simulink model "UR5_simulink"  (R2022b)
settings: Solver=FixedStepAuto  StartTime=0.0  StopTime=8  FixedStep=1e-4  RelTol=1e-3  AbsTol=1e-3  EnableMultiTasking=on
values from neighbouring files (symbols this model uses):
  a1 = 0    [UR5_matlab.m]
  a2 = -0.425    [UR5_matlab.m]
  a3 = -0.39225    [UR5_matlab.m]
  a4 = 0    [UR5_matlab.m]
  a5 = 0    [UR5_matlab.m]
  a6 = 0    [UR5_matlab.m]
  d1 = 0.089159    [UR5_matlab.m]
  d2 = 0    [UR5_matlab.m]
  d3 = 0    [UR5_matlab.m]
  d4 = 0.10915    [UR5_matlab.m]
  d5 = 0.09465    [UR5_matlab.m]
  d6 = 0.0823    [UR5_matlab.m]
  K_fb_1 = fb_action(K1_20,N,Jin_20,Bmw,J1_est,wR1)    [UR5_matlab.m]
  K_fb_2 = fb_action(K1_20,N,Jin_20,Bmw,J2_est,wR2)    [UR5_matlab.m]
  K_fb_3 = fb_action(K1_20,N,Jin_20,Bmw,J3_est,wR3)    [UR5_matlab.m]
  K_fb_4 = fb_action(K1_14,N,Jin_14,Bmw,J4_est,wR4)    [UR5_matlab.m]
  K_fb_5 = fb_action(K1_14,N,Jin_14,Bmw,J5_est,wR5)    [UR5_matlab.m]
  K_fb_6 = fb_action(K1_14,N,Jin_14,Bmw,J6_est,wR6)    [UR5_matlab.m]
  m1 = 3.7    [UR5_matlab.m]
  m2 = 8.393    [UR5_matlab.m]
  m3 = 2.33    [UR5_matlab.m]
  m4 = 1.1219    [UR5_matlab.m]
  m5 = 1.1219    [UR5_matlab.m]
  m6 = 0.1879    [UR5_matlab.m]
  N = 100    [UR5_matlab.m]
undefined symbols (not defined in the file or in its folder): X, Y, Z
libraries: fl_lib x60, sm_lib x33, nesl_utility x31, MyComponent_lib x12
(part 1 of 2)
settings Model: Creator=FrePa  LastModifiedBy=jacop
settings SolverCC: AutoScaleAbsTol=off  AlgebraicLoopSolver=TrustRegion
settings DebuggingCC: UnconnectedInputMsg=warning  UnconnectedOutputMsg=warning  UnconnectedLineMsg=warning  SymbolicDimsDataTypeCodeGenerationDiagnostic=none  SFMachineParentedDataDiag=warning
settings ModelReferenceCC: EnableRefExpFcnMdlSchedulingChecks=on
settings SFSimCC: CustomCodeUndefinedFunction=UseInterfaceOnly
settings RTWCC: DLArmComputeVersion=19.05
settings SimscapeCC: SimscapeLogType=all  SimscapeLogSimulationStatistics=on  SimscapeLogDataHistory=10000
settings ExplorerConfigSet: InternalSimMechanicsExplorerSettings="<ExplorerConfiguration><canonicalview>default</canonicalview><AnimationSetting><BasePlaybackSpeed>1.0</BasePlaybackSpeed><PlaybackSpeedFactor>1.0</PlaybackSpeedFactor></AnimationSetting><TilePanel><TileInfo><Tiles Columns=\"1\" Count=\"1\" Rows=\"1\"><Column Weight=\"1\"/><Row Weight=\"1\"/><Tile Height=\"1\" Width=\"1\" X=\"0\" Y=\"0\"/></Tiles></TileInfo><SceneInfo><SceneViewer><BGColor><R>0.800000011920928955</R><G>0.800000011920928955</G><B>0.800000011920928955</B></BGColor><Camera><DoPerspective>off</DoPerspective><Position><X>-0.833530405890455017</X><Y>-1.17623602270469418</Y><Z>0.420539871522679465</Z></Position><Center><X>0.0136349575198428698</X><Y>0.0260154314115551427</Y><Z>0.247488077140803453</Z></Center><Up><X>0.101701536908081563</X><Y>0.0711627058760085085</Y><Z>0.992266429283455653</Z></Up><ViewLimDist>1</ViewLimDist><YLim>0.821541127691972517</YLim><XLim>1.22120978440698602</XLim></Camera></SceneViewer></SceneInfo></TilePanel><MechEditorPanel><Cameras/><GfxPanelCameraMap/><VideoCreator><PlaybackSpeedRatio>1.0</PlaybackSpeedRatio><FrameRate>30</FrameRate><VideoFormat>Motion JPEG AVI</VideoFormat><FrameSize>auto</FrameSize></VideoCreator></MechEditorPanel></ExplorerConfiguration>"

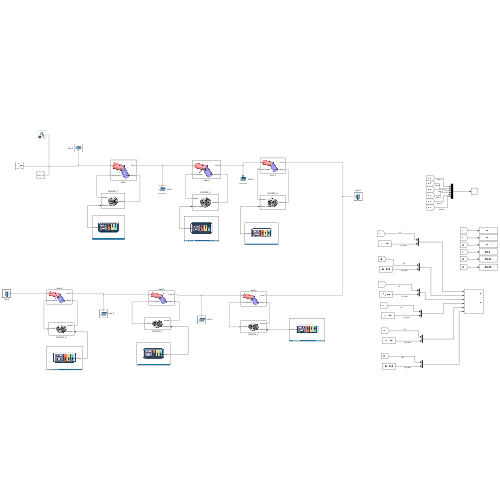
[thumbnail: Simulink's stored preview of the top-level diagram]
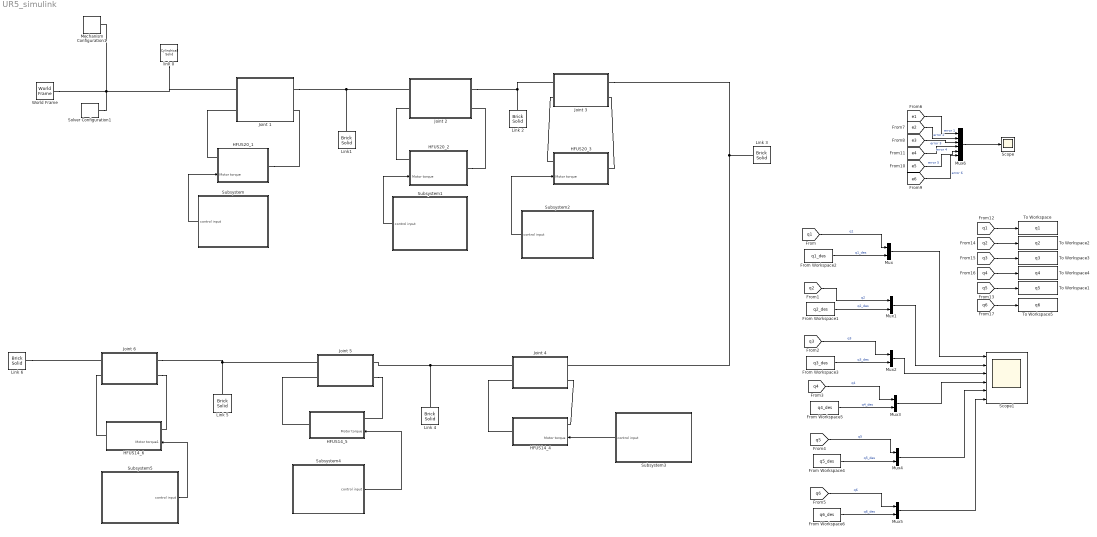
== system UR5_simulink ==
  From Workspace1 : FromWorkspace  VariableName=q2_des
  From Workspace2 : FromWorkspace  VariableName=q1_des
  From Workspace3 : FromWorkspace  VariableName=q3_des
  From Workspace4 : FromWorkspace  VariableName=q5_des
  From Workspace5 : FromWorkspace  VariableName=q4_des
  From Workspace6 : FromWorkspace  VariableName=q6_des
  HFUS14_4 : Subsystem
      settings: PortSchema="{\"entries\":[{\"content\":{\"sides\":[{\"content\":{\"connectorIds\":[\"LConn1\",\"In1\"]},\"type\":\"ConnectorPlacement.EquallySpacedRectSide\",\"uuid\":\"4949b501-9e24-4d03-87d2-659e8cd3beb4\"},{\"content\":{\"connectorIds\":[\"RConn1\"],\"side\":\"RIGHT\"},\"type\":\"ConnectorPlacement.EquallySpacedRectSide\",\"uuid\":\"cef4bc34-d56a-4a9d-a11a-d5ca4c8e0aed\"},{\"content\":{\"connectorIds\":[],\"side\":\"TOP\"},\"type\":\"ConnectorPlacement.EquallySpacedRectSide\",\"uuid\":\"8245fce7-f5cc-4776-a5c0-8930c8ed0033\"}]},\"type\":\"ConnectorPlacement.EquallySpacedConnector\",\"uuid\":\"b9012271-24e3-4605-81e2-55b4e9a8408d\"}],\"packageUris\":[\"http://schema.mathworks.com/mf0/Connector/R2020b\"],\"version\":\"1.0\"}"
      mask Display: image('images.jpeg'); % Use "Edit Image" on toolstrip to change.
  HFUS14_5 : Subsystem
      settings: PortSchema="{\"entries\":[{\"content\":{\"sides\":[{\"content\":{\"connectorIds\":[\"LConn1\",\"In1\"]},\"type\":\"ConnectorPlacement.EquallySpacedRectSide\",\"uuid\":\"4949b501-9e24-4d03-87d2-659e8cd3beb4\"},{\"content\":{\"connectorIds\":[\"RConn1\"],\"side\":\"RIGHT\"},\"type\":\"ConnectorPlacement.EquallySpacedRectSide\",\"uuid\":\"cef4bc34-d56a-4a9d-a11a-d5ca4c8e0aed\"},{\"content\":{\"connectorIds\":[],\"side\":\"TOP\"},\"type\":\"ConnectorPlacement.EquallySpacedRectSide\",\"uuid\":\"8245fce7-f5cc-4776-a5c0-8930c8ed0033\"}]},\"type\":\"ConnectorPlacement.EquallySpacedConnector\",\"uuid\":\"b9012271-24e3-4605-81e2-55b4e9a8408d\"}],\"packageUris\":[\"http://schema.mathworks.com/mf0/Connector/R2020b\"],\"version\":\"1.0\"}"
      mask Display: image('images.jpeg'); % Use "Edit Image" on toolstrip to change.
  HFUS14_6 : Subsystem
      settings: PortSchema="{\"entries\":[{\"content\":{\"sides\":[{\"content\":{\"connectorIds\":[\"LConn1\",\"In1\"]},\"type\":\"ConnectorPlacement.EquallySpacedRectSide\",\"uuid\":\"4949b501-9e24-4d03-87d2-659e8cd3beb4\"},{\"content\":{\"connectorIds\":[\"RConn1\"],\"side\":\"RIGHT\"},\"type\":\"ConnectorPlacement.EquallySpacedRectSide\",\"uuid\":\"cef4bc34-d56a-4a9d-a11a-d5ca4c8e0aed\"},{\"content\":{\"connectorIds\":[],\"side\":\"TOP\"},\"type\":\"ConnectorPlacement.EquallySpacedRectSide\",\"uuid\":\"8245fce7-f5cc-4776-a5c0-8930c8ed0033\"}]},\"type\":\"ConnectorPlacement.EquallySpacedConnector\",\"uuid\":\"b9012271-24e3-4605-81e2-55b4e9a8408d\"}],\"packageUris\":[\"http://schema.mathworks.com/mf0/Connector/R2020b\"],\"version\":\"1.0\"}"
      mask Display: image('images.jpeg'); % Use "Edit Image" on toolstrip to change.
  HFUS20_1 : Subsystem
      settings: PortSchema="{\"entries\":[{\"content\":{\"sides\":[{\"content\":{\"connectorIds\":[\"LConn1\",\"In1\"]},\"type\":\"ConnectorPlacement.EquallySpacedRectSide\",\"uuid\":\"4949b501-9e24-4d03-87d2-659e8cd3beb4\"},{\"content\":{\"connectorIds\":[\"RConn1\"],\"side\":\"RIGHT\"},\"type\":\"ConnectorPlacement.EquallySpacedRectSide\",\"uuid\":\"cef4bc34-d56a-4a9d-a11a-d5ca4c8e0aed\"},{\"content\":{\"connectorIds\":[],\"side\":\"TOP\"},\"type\":\"ConnectorPlacement.EquallySpacedRectSide\",\"uuid\":\"8245fce7-f5cc-4776-a5c0-8930c8ed0033\"}]},\"type\":\"ConnectorPlacement.EquallySpacedConnector\",\"uuid\":\"b9012271-24e3-4605-81e2-55b4e9a8408d\"}],\"packageUris\":[\"http://schema.mathworks.com/mf0/Connector/R2020b\"],\"version\":\"1.0\"}"
      mask Display: image('images.jpeg'); % Use "Edit Image" on toolstrip to change.
  HFUS20_2 : Subsystem
      settings: PortSchema="{\"entries\":[{\"content\":{\"sides\":[{\"content\":{\"connectorIds\":[\"LConn1\",\"In1\"]},\"type\":\"ConnectorPlacement.EquallySpacedRectSide\",\"uuid\":\"4949b501-9e24-4d03-87d2-659e8cd3beb4\"},{\"content\":{\"connectorIds\":[\"RConn1\"],\"side\":\"RIGHT\"},\"type\":\"ConnectorPlacement.EquallySpacedRectSide\",\"uuid\":\"cef4bc34-d56a-4a9d-a11a-d5ca4c8e0aed\"},{\"content\":{\"connectorIds\":[],\"side\":\"TOP\"},\"type\":\"ConnectorPlacement.EquallySpacedRectSide\",\"uuid\":\"8245fce7-f5cc-4776-a5c0-8930c8ed0033\"}]},\"type\":\"ConnectorPlacement.EquallySpacedConnector\",\"uuid\":\"b9012271-24e3-4605-81e2-55b4e9a8408d\"}],\"packageUris\":[\"http://schema.mathworks.com/mf0/Connector/R2020b\"],\"version\":\"1.0\"}"
      mask Display: image('images.jpeg'); % Use "Edit Image" on toolstrip to change.
  HFUS20_3 : Subsystem
      settings: PortSchema="{\"entries\":[{\"content\":{\"sides\":[{\"content\":{\"connectorIds\":[\"LConn1\",\"In1\"]},\"type\":\"ConnectorPlacement.EquallySpacedRectSide\",\"uuid\":\"4949b501-9e24-4d03-87d2-659e8cd3beb4\"},{\"content\":{\"connectorIds\":[\"RConn1\"],\"side\":\"RIGHT\"},\"type\":\"ConnectorPlacement.EquallySpacedRectSide\",\"uuid\":\"cef4bc34-d56a-4a9d-a11a-d5ca4c8e0aed\"},{\"content\":{\"connectorIds\":[],\"side\":\"TOP\"},\"type\":\"ConnectorPlacement.EquallySpacedRectSide\",\"uuid\":\"8245fce7-f5cc-4776-a5c0-8930c8ed0033\"}]},\"type\":\"ConnectorPlacement.EquallySpacedConnector\",\"uuid\":\"b9012271-24e3-4605-81e2-55b4e9a8408d\"}],\"packageUris\":[\"http://schema.mathworks.com/mf0/Connector/R2020b\"],\"version\":\"1.0\"}"
      mask Display: image('images.jpeg'); % Use "Edit Image" on toolstrip to change.
  Joint 1 : Subsystem
      mask Display: image('Revolute-1-DOF-Joint.png'); % Use "Edit Image" on toolstrip to change.
  Joint 2 : Subsystem
      mask Display: image('Revolute-1-DOF-Joint.png'); % Use "Edit Image" on toolstrip to change.
  Joint 3 : Subsystem
      mask Display: image('Revolute-1-DOF-Joint.png'); % Use "Edit Image" on toolstrip to change.
  Joint 4 : Subsystem
      mask Display: image('Revolute-1-DOF-Joint.png'); % Use "Edit Image" on toolstrip to change.
  Joint 5 : Subsystem
      mask Display: image('Revolute-1-DOF-Joint.png'); % Use "Edit Image" on toolstrip to change.
  Joint 6 : Subsystem
      mask Display: image('Revolute-1-DOF-Joint.png'); % Use "Edit Image" on toolstrip to change.
  Link 2 : sm_lib/Body Elements/Brick Solid  GraphicAmbientColor=[0.15 0.15 0.15 1.0]  BasedOnType=Density  BrickDimensions=[1 0.2 0.2]  BrickDimensionUnits=m  CenterOfMass=rG2  CenterOfMassUnits=m  GraphicDiffuseColor=[0.2 0.6 1.0]  Density=1000  DensityUnits=kg/m^3  DoExposeReferenceFrame=on  GraphicEmissiveColor=[0.0 0.0 0.0 1.0]  ExportEntireGeometry=off  SerializedFrames=<Frames/>  MarkerShape=Sphere  MarkerSize=10  GraphicType=FromGeometry  InertiaType=Custom  Mass=m2  MassUnits=kg  MomentsOfInertia=I2  MomentsOfInertiaUnits=kg*m^2  GraphicOpacity=1.0  ProductsOfInertia=[0 0 0]  ProductsOfInertiaUnits=kg*m^2  GraphicShininess=75  GraphicSpecularColor=[0.5 0.5 0.5 1.0]  GraphicVisPropType=SimpleVisualProperties
  Link 3 : sm_lib/Body Elements/Brick Solid  GraphicAmbientColor=[0.15 0.15 0.15 1.0]  BasedOnType=Density  BrickDimensions=[1 0.3 0.2]  BrickDimensionUnits=m  CenterOfMass=rG3  CenterOfMassUnits=m  GraphicDiffuseColor=[0.0 0.8 0.0]  Density=1000  DensityUnits=kg/m^3  DoExposeReferenceFrame=on  GraphicEmissiveColor=[0.0 0.0 0.0 1.0]  ExportEntireGeometry=off  SerializedFrames=<Frames/>  MarkerShape=Sphere  MarkerSize=10  GraphicType=FromGeometry  InertiaType=Custom  Mass=m3  MassUnits=kg  MomentsOfInertia=I3  MomentsOfInertiaUnits=kg*m^2  GraphicOpacity=1.0  ProductsOfInertia=I3_cross  ProductsOfInertiaUnits=kg*m^2  GraphicShininess=75  GraphicSpecularColor=[0.5 0.5 0.5 1.0]  GraphicVisPropType=SimpleVisualProperties
  Link 4 : sm_lib/Body Elements/Brick Solid  GraphicAmbientColor=[0.15 0.15 0.15 1.0]  BasedOnType=Density  BrickDimensions=[0.3 0.3 0.3]  BrickDimensionUnits=m  CenterOfMass=rG4  CenterOfMassUnits=m  GraphicDiffuseColor=[1.0 0.0 0.0]  Density=1000  DensityUnits=kg/m^3  DoExposeReferenceFrame=on  GraphicEmissiveColor=[0.0 0.0 0.0 1.0]  ExportEntireGeometry=off  SerializedFrames=<Frames/>  MarkerShape=Sphere  MarkerSize=10  GraphicType=FromGeometry  InertiaType=Custom  Mass=m4  MassUnits=kg  MomentsOfInertia=I4  MomentsOfInertiaUnits=kg*m^2  GraphicOpacity=1.0  ProductsOfInertia=[0 0 0]  ProductsOfInertiaUnits=kg*m^2  GraphicShininess=75  GraphicSpecularColor=[0.5 0.5 0.5 1.0]  GraphicVisPropType=SimpleVisualProperties
  "Link 5 " : sm_lib/Body Elements/Brick Solid  GraphicAmbientColor=[0.15 0.15 0.15 1.0]  BasedOnType=Density  BrickDimensions=[0.3 0.3 0.3]  BrickDimensionUnits=m  CenterOfMass=rG5  CenterOfMassUnits=m  GraphicDiffuseColor=[0.0 0.0 0.8]  Density=1000  DensityUnits=kg/m^3  DoExposeReferenceFrame=on  GraphicEmissiveColor=[0.0 0.0 0.0 1.0]  ExportEntireGeometry=off  SerializedFrames=<Frames/>  MarkerShape=Sphere  MarkerSize=10  GraphicType=FromGeometry  InertiaType=Custom  Mass=m5  MassUnits=kg  MomentsOfInertia=I5  MomentsOfInertiaUnits=kg*m^2  GraphicOpacity=1.0  ProductsOfInertia=[0 0 0]  ProductsOfInertiaUnits=kg*m^2  GraphicShininess=75  GraphicSpecularColor=[0.5 0.5 0.5 1.0]  GraphicVisPropType=SimpleVisualProperties
  Link 6 : sm_lib/Body Elements/Brick Solid  GraphicAmbientColor=[0.15 0.15 0.15 1.0]  BasedOnType=Density  BrickDimensions=[0.3 0.3 0.3]  BrickDimensionUnits=m  CenterOfMass=rG6  CenterOfMassUnits=m  GraphicDiffuseColor=[0.4 0.4 0.4]  Density=1000  DensityUnits=kg/m^3  DoExposeReferenceFrame=on  GraphicEmissiveColor=[0.0 0.0 0.0 1.0]  ExportEntireGeometry=off  SerializedFrames=<Frames/>  MarkerShape=Sphere  MarkerSize=10  GraphicType=FromGeometry  InertiaType=Custom  Mass=m6  MassUnits=kg  MomentsOfInertia=I6  MomentsOfInertiaUnits=kg*m^2  GraphicOpacity=1.0  ProductsOfInertia=[0 0 0]  ProductsOfInertiaUnits=kg*m^2  GraphicShininess=75  GraphicSpecularColor=[0.5 0.5 0.5 1.0]  GraphicVisPropType=SimpleVisualProperties
  Link1 : sm_lib/Body Elements/Brick Solid  GraphicAmbientColor=[0.15 0.15 0.15 1.0]  BasedOnType=Density  BrickDimensions=[0.2 0.2 0.2]  BrickDimensionUnits=m  CenterOfMass=rG1  CenterOfMassUnits=m  GraphicDiffuseColor=[0.8 0.0 0.4]  Density=1000  DensityUnits=kg/m^3  DoExposeReferenceFrame=on  GraphicEmissiveColor=[0.0 0.0 0.0 1.0]  ExportEntireGeometry=off  SerializedFrames=<Frames/>  MarkerShape=Sphere  MarkerSize=10  GraphicType=FromGeometry  InertiaType=Custom  Mass=m1  MassUnits=kg  MomentsOfInertia=I1  MomentsOfInertiaUnits=kg*m^2  GraphicOpacity=1.0  ProductsOfInertia=[0 0 0]  ProductsOfInertiaUnits=kg*m^2  GraphicShininess=75  GraphicSpecularColor=[0.5 0.5 0.5 1.0]  GraphicVisPropType=SimpleVisualProperties
  Mechanism Configuration1 : sm_lib/Utilities/Mechanism Configuration  UniformGravity=Constant  GravityVector=[0 0 -9.80665]  GravityUnits=m/s^2  LinearizationDelta=0.001  JointModeTransitionNonlinearIterations=2
  Mux{,1..5} (6 alike) : Mux  Inputs=2
  Mux6 : Mux  Inputs=6
  Scope : Scope
  Scope1 : Scope  NumInputPorts=6
  Solver Configuration1 : nesl_utility/Solver Configuration  PhysicalDomain=network_engine_domain  SubClassName=solver  LeftPortType=input  RightPortType=generic  Tones=[]  Harmonics=[]  SimulateNoise=off  Profile=off  UseLocalSampling=off  EnableSwitchedLinearOptims=on  FrequencyDomain=off  UseCCode=off  RelTol=0.001  AbsTol=1e-06  MinStep=1e-09  ToWorkspace=off  RevertToSquareIcSolve=off  NumHomotopyIterations=100  PhasorMode=off  PhasorModeNumHarmonics=1  ConsistencySolver=NEWTON_XTOL_AFTER_FTOL  IndexReductionMethod=DerivativeReplacement  DoDC=off  ResidualTolerance=1e-09  ConsistencyTolSource=GLOBAL  ConsistencyAbsTol=0.001  ConsistencyRelTol=0.001  ConsistencyTolFactor=0.001  UseLocalSolver=off  LocalSolverChoice=NE_BACKWARD_EULER_ADVANCER  ResolveIndetEquations=on  FunctionEvalNumThread=1  LocalSolverSampleTime=0.001  DoFixedCost=off  MaxNonlinIter=3  MaxModeIter=2  ComputeImpulses=off  ImpulseIterations=2  LinearAlgebra=Sparse  LinearAlgebraNumThread=0  EquationFormulation=NE_TIME_EF  DelaysMemoryBudget=1024  AutomaticFiltering=on  FilteringTimeConstant=0.001  PartitionStorageMethod=AS_NEEDED  PartitionMemoryBudget=1024  PartitionMethod=FAST
  Subsystem : Subsystem
      mask Display: image('images.png'); % Use "Edit Image" on toolstrip to change.
  Subsystem1 : Subsystem
      mask Display: image('images.png'); % Use "Edit Image" on toolstrip to change.
  Subsystem2 : Subsystem
      mask Display: image('images.png'); % Use "Edit Image" on toolstrip to change.
  Subsystem3 : Subsystem
      mask Display: image('images.png'); % Use "Edit Image" on toolstrip to change.
  Subsystem4 : Subsystem
      mask Display: image('images.png'); % Use "Edit Image" on toolstrip to change.
  Subsystem5 : Subsystem
      mask Display: image('images.png'); % Use "Edit Image" on toolstrip to change.
  To Workspace : ToWorkspace  VariableName=q1  SaveFormat=Timeseries  SampleTime=-1
  To Workspace1 : ToWorkspace  VariableName=q5  SaveFormat=Timeseries  SampleTime=-1
  To Workspace2 : ToWorkspace  VariableName=q2  SaveFormat=Timeseries  SampleTime=-1
  To Workspace3 : ToWorkspace  VariableName=q3  SaveFormat=Timeseries  SampleTime=-1
  To Workspace4 : ToWorkspace  VariableName=q4  SaveFormat=Timeseries  SampleTime=-1
  To Workspace5 : ToWorkspace  VariableName=q6  SaveFormat=Timeseries  SampleTime=-1
  World Frame : sm_lib/Frames and Transforms/World Frame
  link 0 : sm_lib/Body Elements/Cylindrical Solid  GraphicAmbientColor=[0.15 0.15 0.15 1.0]  BasedOnType=Density  CenterOfMass=[0 0 0]  CenterOfMassUnits=m  GraphicDiffuseColor=[0.5 0.5 0.5]  CylinderLength=0.05  CylinderLengthUnits=m  CylinderRadius=1  CylinderRadiusUnits=m  Density=1000  DensityUnits=kg/m^3  DoExposeReferenceFrame=on  GraphicEmissiveColor=[0.0 0.0 0.0 1.0]  ExportEntireGeometry=off  SerializedFrames=<Frames/>  MarkerShape=Sphere  MarkerSize=10  GraphicType=FromGeometry  InertiaType=Custom  Mass=m1  MassUnits=kg  MomentsOfInertia=I1  MomentsOfInertiaUnits=kg*m^2  GraphicOpacity=1.0  ProductsOfInertia=[0 0 0]  ProductsOfInertiaUnits=kg*m^2  GraphicShininess=75  GraphicSpecularColor=[0.5 0.5 0.5 1.0]  GraphicVisPropType=SimpleVisualProperties
  wires:
  Subsystem1/1("control input ") -> HFUS20_2/1(Motor torque)
  Subsystem2/1("control input ") -> HFUS20_3/1(Motor torque)
  Subsystem3/1("control input ") -> HFUS14_4/1(Motor torque)
  Subsystem5/1("control input ") -> HFUS14_6/1(Motor torque1)
  Subsystem4/1("control input ") -> HFUS14_5/1(Motor torque)
  Subsystem/1("control input ") -> HFUS20_1/1(Motor torque)
  From Workspace2/1 -> Mux/2  "q1_des"
  [q1] -> Mux/1  "q1"
  [q2] -> Mux1/1  "q2"
  From Workspace1/1 -> Mux1/2  "q2_des"
  [q3] -> Mux2/1  "q3"
  From Workspace3/1 -> Mux2/2  "q3_des"
  Mux/1 -> Scope1/1
  [q4] -> Mux3/1  "q4"
  From Workspace5/1 -> Mux3/2  "q4_des"
  [q6] -> Mux5/1  "q6"
  From Workspace4/1 -> Mux4/2  "q5_des"
  From Workspace6/1 -> Mux5/2  "q6_des"
  [q5] -> Mux4/1  "q5"
  Mux1/1 -> Scope1/2
  Mux2/1 -> Scope1/3
  Mux3/1 -> Scope1/4
  Mux4/1 -> Scope1/5
  Mux5/1 -> Scope1/6
  [e1] -> Mux6/1  "error 1"
  [e2] -> Mux6/2  "error 2"
  [e3] -> Mux6/3  "error 3"
  [e4] -> Mux6/4  "error 4"
  [e5] -> Mux6/5  "error 5"
  [e6] -> Mux6/6  "error 6"
  Mux6/1 -> Scope/1
  [q1] -> To Workspace/1
  [q5] -> To Workspace1/1
  [q2] -> To Workspace2/1
  [q3] -> To Workspace3/1
  [q4] -> To Workspace4/1
  [q6] -> To Workspace5/1
  connections:
  Joint 1/RConn1 -- Link1/RConn1 -- Joint 2/LConn1
  Joint 3/RConn1 -- Joint 4/LConn1 -- Link 3/RConn1
  Joint 4/RConn1 -- Link 4/RConn1 -- Joint 5/LConn2
  Joint 6/LConn1 -- "Link 5 "/RConn1 -- Joint 5/RConn2
  Link 6/RConn1 -- Joint 6/RConn1
  World Frame/RConn1 -- Joint 1/LConn1 -- link 0/RConn1 -- Mechanism Configuration1/RConn1 -- Solver Configuration1/RConn1
  Joint 2/RConn1 -- Link 2/RConn1 -- Joint 3/LConn1
  HFUS20_1/RConn1 -- Joint 1/RConn2
  Joint 2/LConn2 -- HFUS20_2/LConn1
  HFUS20_2/RConn1 -- Joint 2/RConn2
  HFUS20_3/RConn1 -- Joint 3/RConn2
  HFUS20_3/LConn1 -- Joint 3/LConn2
  Joint 4/LConn2 -- HFUS14_4/LConn1
  Joint 4/RConn2 -- HFUS14_4/RConn1
  HFUS14_6/RConn1 -- Joint 6/RConn2
  Joint 6/LConn2 -- HFUS14_6/LConn1
  HFUS14_5/RConn1 -- Joint 5/RConn1
  Joint 5/LConn1 -- HFUS14_5/LConn1
  HFUS20_1/LConn1 -- Joint 1/LConn2

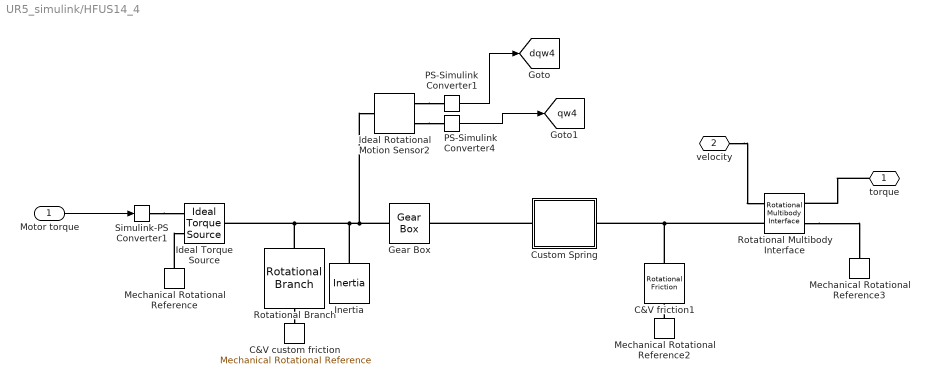
== system UR5_simulink/HFUS14_4 ==
  Motor torque : Inport
  C&V custom friction : fl_lib/Mechanical/Rotational Elements/Mechanical Rotational Reference
  C&V friction1 : fl_lib/Mechanical/Rotational Elements/Rotational Friction  brkwy_trq=0.4 N*m  brkwy_vel=0.1 rad/s  Col_trq=Bf_plus N*m  visc_coef=0 N*m*s/rad  w_specify=off  w_priority=None  w=0 rad/s  w_nominal_specify=off  w_nominal_unit=rad/s  w_nominal_value=1  t_specify=off  t_priority=None  t=0 N*m  t_nominal_specify=off  t_nominal_unit=N*m  t_nominal_value=1
  Custom Spring : Subsystem
      mask Display: image('C:\Users\laura\OneDrive\Desktop\download.jpeg'); % Use "Edit Image" on toolstrip to change.
  Gear Box : fl_lib/Mechanical/Mechanisms/Gear Box  ratio=N  t_in_specify=off  t_in_priority=None  t_in=0 N*m  t_in_nominal_specify=off  t_in_nominal_unit=N*m  t_in_nominal_value=1  t_out_specify=off  t_out_priority=None  t_out=0 N*m  t_out_nominal_specify=off  t_out_nominal_unit=N*m  t_out_nominal_value=1
  Ideal Rotational Motion Sensor2 : fl_lib/Mechanical/Mechanical Sensors/Ideal Rotational Motion Sensor  reference=foundation.enum.MeasurementReference.absolute  acceleration_port=false  velocity_port=true  position_port=true  wrap_angle=false  offset=0 rad
      settings: InternalSimscapePortConfiguration="{\"Bottom\":[],\"Left\":[{\"id\":\"R\",\"label\":\"R\",\"type\":\"foundation.mechanical.rotational.rotational\"}],\"Right\":[{\"id\":\"W\",\"label\":\"W\",\"type\":\"output\"},{\"id\":\"A\",\"label\":\"A\",\"type\":\"output\"}],\"Top\":[]}"
  Ideal Torque Source : fl_lib/Mechanical/Mechanical Sources/Ideal Torque Source
  Inertia : fl_lib/Mechanical/Rotational Elements/Inertia  inertia=Jin_14 kg*m^2  num_ports=foundation.enum.numPorts2.one  w_specify=off  w_priority=High  w=0 rad/s  w_nominal_specify=off  w_nominal_unit=rad/s  w_nominal_value=1  t_specify=off  t_priority=None  t=0 N*m  t_nominal_specify=off  t_nominal_unit=N*m  t_nominal_value=1
  Mechanical Rotational Reference : fl_lib/Mechanical/Rotational Elements/Mechanical Rotational Reference
  Mechanical Rotational Reference2 : fl_lib/Mechanical/Rotational Elements/Mechanical Rotational Reference
  Mechanical Rotational Reference3 : fl_lib/Mechanical/Rotational Elements/Mechanical Rotational Reference
  PS-Simulink Converter1 : nesl_utility/PS-Simulink Converter  PhysicalDomain=network_engine_domain  SubClassName=ps_output  LeftPortType=input  RightPortType=output  PseudoPeriodic=off  Frequencies=[]  VectorFormat=inherit  Unit=inherit  AffineConversion=off
  PS-Simulink Converter4 : nesl_utility/PS-Simulink Converter  PhysicalDomain=network_engine_domain  SubClassName=ps_output  LeftPortType=input  RightPortType=output  PseudoPeriodic=off  Frequencies=[]  VectorFormat=inherit  Unit=inherit  AffineConversion=off
  Rotational Branch : MyComponent_lib/Rotational Branch  brkwy_trq=25 N*m  brkwy_vel=0.1 rad/s  Col_trq_p=0.008 N*m  Col_trq_m=-0.007 N*m  visc_coef=6.4e-4 N*m*s/rad  w_specify=off  w_priority=None  w=0 rad/s  w_nominal_specify=off  w_nominal_unit=rad/s  w_nominal_value=1  t_specify=off  t_priority=None  t=0 N*m  t_nominal_specify=off  t_nominal_unit=N*m  t_nominal_value=1
      settings: InternalSimscapePortConfiguration="{\"Bottom\":[],\"Left\":[{\"id\":\"R\",\"label\":\"R\",\"type\":\"foundation.mechanical.rotational.rotational\"}],\"Right\":[{\"id\":\"C\",\"label\":\"C\",\"type\":\"foundation.mechanical.rotational.rotational\"}],\"Top\":[]}"
  Rotational Multibody Interface : fl_lib/Mechanical/Multibody Interfaces/Rotational Multibody Interface
  Simulink-PS Converter1 : nesl_utility/Simulink-PS Converter  PhysicalDomain=network_engine_domain  SubClassName=ps_input  LeftPortType=input  RightPortType=output  PseudoPeriodic=off  Frequencies=[]  NoiseDistribution=none  NoiseParameters=[]  Unit=1  AffineConversion=off  FilteringAndDerivatives=provide  SimscapeFilterOrder=1  InputFilterTimeConstant=0.001  UdotUserProvided=0
  torque : PMIOPort  Side=Left
  velocity : PMIOPort  Port=2  Side=Right
  tag scope: dqw4=global, qw4=global
  wires:
  Motor torque/1 -> Simulink-PS Converter1/1
  PS-Simulink Converter4/1 -> [qw4]
  PS-Simulink Converter1/1 -> [dqw4]
  connections:
  Simulink-PS Converter1/RConn1 -- Ideal Torque Source/RConn1
  Mechanical Rotational Reference/LConn1 -- Ideal Torque Source/RConn2
  Ideal Rotational Motion Sensor2/LConn1 -- Gear Box/LConn1 -- Inertia/LConn1 -- Rotational Branch/LConn1 -- Ideal Torque Source/LConn1
  velocity/RConn1 -- Rotational Multibody Interface/RConn1
  torque/RConn1 -- Rotational Multibody Interface/LConn1
  Custom Spring/LConn1 -- Gear Box/RConn1
  Ideal Rotational Motion Sensor2/RConn1 -- PS-Simulink Converter1/LConn1
  Ideal Rotational Motion Sensor2/RConn2 -- PS-Simulink Converter4/LConn1
  Rotational Multibody Interface/LConn2 -- Mechanical Rotational Reference3/LConn1
  Rotational Multibody Interface/RConn2 -- Custom Spring/RConn1 -- C&V friction1/LConn1
  Mechanical Rotational Reference2/LConn1 -- C&V friction1/RConn1
  Rotational Branch/RConn1 -- C&V custom friction/LConn1

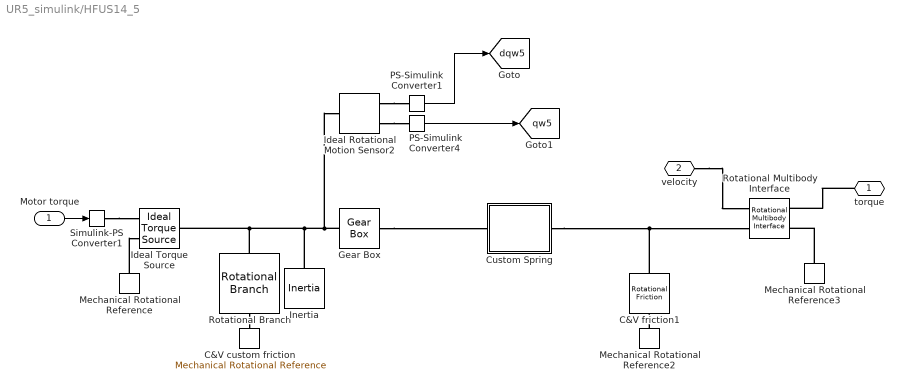
== system UR5_simulink/HFUS14_5 ==
  Motor torque : Inport
  C&V custom friction : fl_lib/Mechanical/Rotational Elements/Mechanical Rotational Reference
  C&V friction1 : fl_lib/Mechanical/Rotational Elements/Rotational Friction  brkwy_trq=0.4 N*m  brkwy_vel=0.1 rad/s  Col_trq=Bf_plus N*m  visc_coef=0 N*m*s/rad  w_specify=off  w_priority=None  w=0 rad/s  w_nominal_specify=off  w_nominal_unit=rad/s  w_nominal_value=1  t_specify=off  t_priority=None  t=0 N*m  t_nominal_specify=off  t_nominal_unit=N*m  t_nominal_value=1
  Custom Spring : Subsystem
      mask Display: image('C:\Users\laura\OneDrive\Desktop\download.jpeg'); % Use "Edit Image" on toolstrip to change.
  Gear Box : fl_lib/Mechanical/Mechanisms/Gear Box  ratio=N  t_in_specify=off  t_in_priority=None  t_in=0 N*m  t_in_nominal_specify=off  t_in_nominal_unit=N*m  t_in_nominal_value=1  t_out_specify=off  t_out_priority=None  t_out=0 N*m  t_out_nominal_specify=off  t_out_nominal_unit=N*m  t_out_nominal_value=1
  Ideal Rotational Motion Sensor2 : fl_lib/Mechanical/Mechanical Sensors/Ideal Rotational Motion Sensor  reference=foundation.enum.MeasurementReference.absolute  acceleration_port=false  velocity_port=true  position_port=true  wrap_angle=false  offset=0 rad
      settings: InternalSimscapePortConfiguration="{\"Bottom\":[],\"Left\":[{\"id\":\"R\",\"label\":\"R\",\"type\":\"foundation.mechanical.rotational.rotational\"}],\"Right\":[{\"id\":\"W\",\"label\":\"W\",\"type\":\"output\"},{\"id\":\"A\",\"label\":\"A\",\"type\":\"output\"}],\"Top\":[]}"
  Ideal Torque Source : fl_lib/Mechanical/Mechanical Sources/Ideal Torque Source
  Inertia : fl_lib/Mechanical/Rotational Elements/Inertia  inertia=Jin_14 kg*m^2  num_ports=foundation.enum.numPorts2.one  w_specify=off  w_priority=High  w=0 rad/s  w_nominal_specify=off  w_nominal_unit=rad/s  w_nominal_value=1  t_specify=off  t_priority=None  t=0 N*m  t_nominal_specify=off  t_nominal_unit=N*m  t_nominal_value=1
  Mechanical Rotational Reference : fl_lib/Mechanical/Rotational Elements/Mechanical Rotational Reference
  Mechanical Rotational Reference2 : fl_lib/Mechanical/Rotational Elements/Mechanical Rotational Reference
  Mechanical Rotational Reference3 : fl_lib/Mechanical/Rotational Elements/Mechanical Rotational Reference
  PS-Simulink Converter1 : nesl_utility/PS-Simulink Converter  PhysicalDomain=network_engine_domain  SubClassName=ps_output  LeftPortType=input  RightPortType=output  PseudoPeriodic=off  Frequencies=[]  VectorFormat=inherit  Unit=inherit  AffineConversion=off
  PS-Simulink Converter4 : nesl_utility/PS-Simulink Converter  PhysicalDomain=network_engine_domain  SubClassName=ps_output  LeftPortType=input  RightPortType=output  PseudoPeriodic=off  Frequencies=[]  VectorFormat=inherit  Unit=inherit  AffineConversion=off
  Rotational Branch : MyComponent_lib/Rotational Branch  brkwy_trq=25 N*m  brkwy_vel=0.1 rad/s  Col_trq_p=0.008 N*m  Col_trq_m=-0.007 N*m  visc_coef=6.4e-4 N*m*s/rad  w_specify=off  w_priority=None  w=0 rad/s  w_nominal_specify=off  w_nominal_unit=rad/s  w_nominal_value=1  t_specify=off  t_priority=None  t=0 N*m  t_nominal_specify=off  t_nominal_unit=N*m  t_nominal_value=1
      settings: InternalSimscapePortConfiguration="{\"Bottom\":[],\"Left\":[{\"id\":\"R\",\"label\":\"R\",\"type\":\"foundation.mechanical.rotational.rotational\"}],\"Right\":[{\"id\":\"C\",\"label\":\"C\",\"type\":\"foundation.mechanical.rotational.rotational\"}],\"Top\":[]}"
  Rotational Multibody Interface : fl_lib/Mechanical/Multibody Interfaces/Rotational Multibody Interface
  Simulink-PS Converter1 : nesl_utility/Simulink-PS Converter  PhysicalDomain=network_engine_domain  SubClassName=ps_input  LeftPortType=input  RightPortType=output  PseudoPeriodic=off  Frequencies=[]  NoiseDistribution=none  NoiseParameters=[]  Unit=1  AffineConversion=off  FilteringAndDerivatives=provide  SimscapeFilterOrder=1  InputFilterTimeConstant=0.001  UdotUserProvided=0
  torque : PMIOPort  Side=Left
  velocity : PMIOPort  Port=2  Side=Right
  tag scope: dqw5=global, qw5=global
  wires:
  Motor torque/1 -> Simulink-PS Converter1/1
  PS-Simulink Converter4/1 -> [qw5]
  PS-Simulink Converter1/1 -> [dqw5]
  connections:
  Simulink-PS Converter1/RConn1 -- Ideal Torque Source/RConn1
  Mechanical Rotational Reference/LConn1 -- Ideal Torque Source/RConn2
  Ideal Rotational Motion Sensor2/LConn1 -- Gear Box/LConn1 -- Inertia/LConn1 -- Rotational Branch/LConn1 -- Ideal Torque Source/LConn1
  velocity/RConn1 -- Rotational Multibody Interface/RConn1
  torque/RConn1 -- Rotational Multibody Interface/LConn1
  Gear Box/RConn1 -- Custom Spring/LConn1
  Ideal Rotational Motion Sensor2/RConn1 -- PS-Simulink Converter1/LConn1
  Ideal Rotational Motion Sensor2/RConn2 -- PS-Simulink Converter4/LConn1
  Mechanical Rotational Reference3/LConn1 -- Rotational Multibody Interface/LConn2
  Custom Spring/RConn1 -- C&V friction1/LConn1 -- Rotational Multibody Interface/RConn2
  Mechanical Rotational Reference2/LConn1 -- C&V friction1/RConn1
  Rotational Branch/RConn1 -- C&V custom friction/LConn1

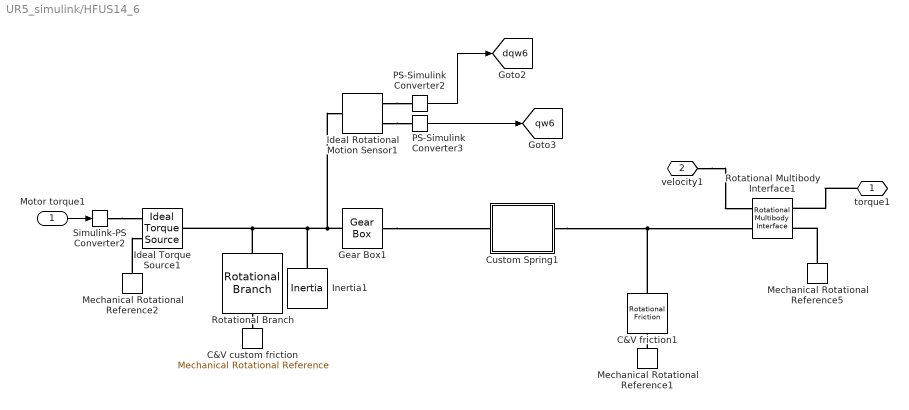
== system UR5_simulink/HFUS14_6 ==
  Motor torque1 : Inport
  C&V custom friction : fl_lib/Mechanical/Rotational Elements/Mechanical Rotational Reference
  C&V friction1 : fl_lib/Mechanical/Rotational Elements/Rotational Friction  brkwy_trq=0.4 N*m  brkwy_vel=0.1 rad/s  Col_trq=Bf_plus N*m  visc_coef=0 N*m*s/rad  w_specify=off  w_priority=None  w=0 rad/s  w_nominal_specify=off  w_nominal_unit=rad/s  w_nominal_value=1  t_specify=off  t_priority=None  t=0 N*m  t_nominal_specify=off  t_nominal_unit=N*m  t_nominal_value=1
  Custom Spring1 : Subsystem
      mask Display: image('C:\Users\laura\OneDrive\Desktop\download.jpeg'); % Use "Edit Image" on toolstrip to change.
  Gear Box1 : fl_lib/Mechanical/Mechanisms/Gear Box  ratio=N  t_in_specify=off  t_in_priority=None  t_in=0 N*m  t_in_nominal_specify=off  t_in_nominal_unit=N*m  t_in_nominal_value=1  t_out_specify=off  t_out_priority=None  t_out=0 N*m  t_out_nominal_specify=off  t_out_nominal_unit=N*m  t_out_nominal_value=1
  Ideal Rotational Motion Sensor1 : fl_lib/Mechanical/Mechanical Sensors/Ideal Rotational Motion Sensor  reference=foundation.enum.MeasurementReference.absolute  acceleration_port=false  velocity_port=true  position_port=true  wrap_angle=false  offset=0 rad
      settings: InternalSimscapePortConfiguration="{\"Bottom\":[],\"Left\":[{\"id\":\"R\",\"label\":\"R\",\"type\":\"foundation.mechanical.rotational.rotational\"}],\"Right\":[{\"id\":\"W\",\"label\":\"W\",\"type\":\"output\"},{\"id\":\"A\",\"label\":\"A\",\"type\":\"output\"}],\"Top\":[]}"
  Ideal Torque Source1 : fl_lib/Mechanical/Mechanical Sources/Ideal Torque Source
  Inertia1 : fl_lib/Mechanical/Rotational Elements/Inertia  inertia=Jin_14 kg*m^2  num_ports=foundation.enum.numPorts2.one  w_specify=off  w_priority=High  w=0 rad/s  w_nominal_specify=off  w_nominal_unit=rad/s  w_nominal_value=1  t_specify=off  t_priority=None  t=0 N*m  t_nominal_specify=off  t_nominal_unit=N*m  t_nominal_value=1
  Mechanical Rotational Reference1 : fl_lib/Mechanical/Rotational Elements/Mechanical Rotational Reference
  Mechanical Rotational Reference2 : fl_lib/Mechanical/Rotational Elements/Mechanical Rotational Reference
  Mechanical Rotational Reference5 : fl_lib/Mechanical/Rotational Elements/Mechanical Rotational Reference
  PS-Simulink Converter2 : nesl_utility/PS-Simulink Converter  PhysicalDomain=network_engine_domain  SubClassName=ps_output  LeftPortType=input  RightPortType=output  PseudoPeriodic=off  Frequencies=[]  VectorFormat=inherit  Unit=inherit  AffineConversion=off
  PS-Simulink Converter3 : nesl_utility/PS-Simulink Converter  PhysicalDomain=network_engine_domain  SubClassName=ps_output  LeftPortType=input  RightPortType=output  PseudoPeriodic=off  Frequencies=[]  VectorFormat=inherit  Unit=inherit  AffineConversion=off
  Rotational Branch : MyComponent_lib/Rotational Branch  brkwy_trq=25 N*m  brkwy_vel=0.1 rad/s  Col_trq_p=0.008 N*m  Col_trq_m=-0.007 N*m  visc_coef=6.4e-4 N*m*s/rad  w_specify=off  w_priority=None  w=0 rad/s  w_nominal_specify=off  w_nominal_unit=rad/s  w_nominal_value=1  t_specify=off  t_priority=None  t=0 N*m  t_nominal_specify=off  t_nominal_unit=N*m  t_nominal_value=1
      settings: InternalSimscapePortConfiguration="{\"Bottom\":[],\"Left\":[{\"id\":\"R\",\"label\":\"R\",\"type\":\"foundation.mechanical.rotational.rotational\"}],\"Right\":[{\"id\":\"C\",\"label\":\"C\",\"type\":\"foundation.mechanical.rotational.rotational\"}],\"Top\":[]}"
  Rotational Multibody Interface1 : fl_lib/Mechanical/Multibody Interfaces/Rotational Multibody Interface
  Simulink-PS Converter2 : nesl_utility/Simulink-PS Converter  PhysicalDomain=network_engine_domain  SubClassName=ps_input  LeftPortType=input  RightPortType=output  PseudoPeriodic=off  Frequencies=[]  NoiseDistribution=none  NoiseParameters=[]  Unit=1  AffineConversion=off  FilteringAndDerivatives=provide  SimscapeFilterOrder=1  InputFilterTimeConstant=0.001  UdotUserProvided=0
  torque1 : PMIOPort  Side=Left
  velocity1 : PMIOPort  Port=2  Side=Right
  tag scope: dqw6=global, qw6=global
  wires:
  PS-Simulink Converter2/1 -> [dqw6]
  PS-Simulink Converter3/1 -> [qw6]
  Motor torque1/1 -> Simulink-PS Converter2/1
  connections:
  Ideal Torque Source1/LConn1 -- Rotational Branch/LConn1 -- Ideal Rotational Motion Sensor1/LConn1 -- Gear Box1/LConn1 -- Inertia1/LConn1
  Ideal Rotational Motion Sensor1/RConn1 -- PS-Simulink Converter2/LConn1
  Mechanical Rotational Reference5/LConn1 -- Rotational Multibody Interface1/LConn2
  Ideal Rotational Motion Sensor1/RConn2 -- PS-Simulink Converter3/LConn1
  velocity1/RConn1 -- Rotational Multibody Interface1/RConn1
  Custom Spring1/RConn1 -- C&V friction1/LConn1 -- Rotational Multibody Interface1/RConn2
  Mechanical Rotational Reference2/LConn1 -- Ideal Torque Source1/RConn2
  Simulink-PS Converter2/RConn1 -- Ideal Torque Source1/RConn1
  torque1/RConn1 -- Rotational Multibody Interface1/LConn1
  Gear Box1/RConn1 -- Custom Spring1/LConn1
  Mechanical Rotational Reference1/LConn1 -- C&V friction1/RConn1
  Rotational Branch/RConn1 -- C&V custom friction/LConn1

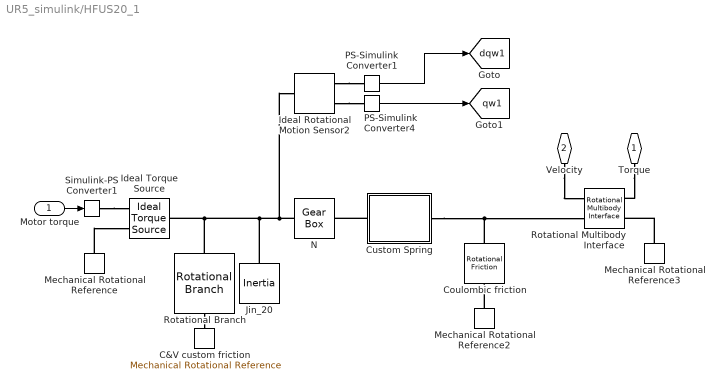
== system UR5_simulink/HFUS20_1 ==
  Motor torque : Inport
  C&V custom friction : fl_lib/Mechanical/Rotational Elements/Mechanical Rotational Reference
  "Coulombic friction " : fl_lib/Mechanical/Rotational Elements/Rotational Friction  brkwy_trq=0.4 N*m  brkwy_vel=0.1 rad/s  Col_trq=Bf_plus N*m  visc_coef=0 N*m*s/rad  w_specify=off  w_priority=None  w=0 rad/s  w_nominal_specify=off  w_nominal_unit=rad/s  w_nominal_value=1  t_specify=off  t_priority=None  t=0 N*m  t_nominal_specify=off  t_nominal_unit=N*m  t_nominal_value=1
  Custom Spring : Subsystem
      mask Display: image('C:\Users\laura\OneDrive\Desktop\download.jpeg'); % Use "Edit Image" on toolstrip to change.
  Ideal Rotational Motion Sensor2 : fl_lib/Mechanical/Mechanical Sensors/Ideal Rotational Motion Sensor  reference=foundation.enum.MeasurementReference.absolute  acceleration_port=false  velocity_port=true  position_port=true  wrap_angle=false  offset=0 rad
      settings: InternalSimscapePortConfiguration="{\"Bottom\":[],\"Left\":[{\"id\":\"R\",\"label\":\"R\",\"type\":\"foundation.mechanical.rotational.rotational\"}],\"Right\":[{\"id\":\"W\",\"label\":\"W\",\"type\":\"output\"},{\"id\":\"A\",\"label\":\"A\",\"type\":\"output\"}],\"Top\":[]}"
  Ideal Torque Source : fl_lib/Mechanical/Mechanical Sources/Ideal Torque Source
  Jin_20 : fl_lib/Mechanical/Rotational Elements/Inertia  inertia=Jin_20 kg*m^2  num_ports=foundation.enum.numPorts2.one  w_specify=off  w_priority=High  w=0 rad/s  w_nominal_specify=off  w_nominal_unit=rad/s  w_nominal_value=1  t_specify=off  t_priority=None  t=0 N*m  t_nominal_specify=off  t_nominal_unit=N*m  t_nominal_value=1
  Mechanical Rotational Reference : fl_lib/Mechanical/Rotational Elements/Mechanical Rotational Reference
  Mechanical Rotational Reference2 : fl_lib/Mechanical/Rotational Elements/Mechanical Rotational Reference
  Mechanical Rotational Reference3 : fl_lib/Mechanical/Rotational Elements/Mechanical Rotational Reference
  N : fl_lib/Mechanical/Mechanisms/Gear Box  ratio=N  t_in_specify=off  t_in_priority=None  t_in=0 N*m  t_in_nominal_specify=off  t_in_nominal_unit=N*m  t_in_nominal_value=1  t_out_specify=off  t_out_priority=None  t_out=0 N*m  t_out_nominal_specify=off  t_out_nominal_unit=N*m  t_out_nominal_value=1
  PS-Simulink Converter1 : nesl_utility/PS-Simulink Converter  PhysicalDomain=network_engine_domain  SubClassName=ps_output  LeftPortType=input  RightPortType=output  PseudoPeriodic=off  Frequencies=[]  VectorFormat=inherit  Unit=inherit  AffineConversion=off
  PS-Simulink Converter4 : nesl_utility/PS-Simulink Converter  PhysicalDomain=network_engine_domain  SubClassName=ps_output  LeftPortType=input  RightPortType=output  PseudoPeriodic=off  Frequencies=[]  VectorFormat=inherit  Unit=inherit  AffineConversion=off
  Rotational Branch : MyComponent_lib/Rotational Branch  brkwy_trq=25 N*m  brkwy_vel=0.1 rad/s  Col_trq_p=0.008 N*m  Col_trq_m=-0.007 N*m  visc_coef=6.4e-4 N*m*s/rad  w_specify=off  w_priority=None  w=0 rad/s  w_nominal_specify=off  w_nominal_unit=rad/s  w_nominal_value=1  t_specify=off  t_priority=None  t=0 N*m  t_nominal_specify=off  t_nominal_unit=N*m  t_nominal_value=1
      settings: InternalSimscapePortConfiguration="{\"Bottom\":[],\"Left\":[{\"id\":\"R\",\"label\":\"R\",\"type\":\"foundation.mechanical.rotational.rotational\"}],\"Right\":[{\"id\":\"C\",\"label\":\"C\",\"type\":\"foundation.mechanical.rotational.rotational\"}],\"Top\":[]}"
  Rotational Multibody Interface : fl_lib/Mechanical/Multibody Interfaces/Rotational Multibody Interface
  Simulink-PS Converter1 : nesl_utility/Simulink-PS Converter  PhysicalDomain=network_engine_domain  SubClassName=ps_input  LeftPortType=input  RightPortType=output  PseudoPeriodic=off  Frequencies=[]  NoiseDistribution=none  NoiseParameters=[]  Unit=1  AffineConversion=off  FilteringAndDerivatives=provide  SimscapeFilterOrder=1  InputFilterTimeConstant=0.001  UdotUserProvided=0
  Torque : PMIOPort  Side=Left
  Velocity : PMIOPort  Port=2  Side=Right
  tag scope: dqw1=global, qw1=global
  wires:
  Motor torque/1 -> Simulink-PS Converter1/1
  PS-Simulink Converter1/1 -> [dqw1]
  PS-Simulink Converter4/1 -> [qw1]
  connections:
  Custom Spring/RConn1 -- Rotational Multibody Interface/RConn2 -- "Coulombic friction "/LConn1
  Simulink-PS Converter1/RConn1 -- Ideal Torque Source/RConn1
  Mechanical Rotational Reference/LConn1 -- Ideal Torque Source/RConn2
  N/LConn1 -- Ideal Rotational Motion Sensor2/LConn1 -- Rotational Branch/LConn1 -- Ideal Torque Source/LConn1 -- Jin_20/LConn1
  Rotational Branch/RConn1 -- C&V custom friction/LConn1
  Velocity/RConn1 -- Rotational Multibody Interface/RConn1
  Torque/RConn1 -- Rotational Multibody Interface/LConn1
  Custom Spring/LConn1 -- N/RConn1
  Mechanical Rotational Reference3/LConn1 -- Rotational Multibody Interface/LConn2
  Mechanical Rotational Reference2/LConn1 -- "Coulombic friction "/RConn1
  Ideal Rotational Motion Sensor2/RConn1 -- PS-Simulink Converter1/LConn1
  Ideal Rotational Motion Sensor2/RConn2 -- PS-Simulink Converter4/LConn1

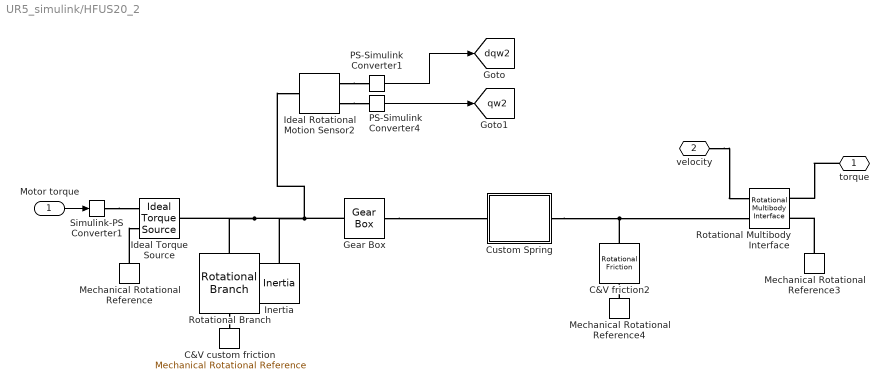
== system UR5_simulink/HFUS20_2 ==
  Motor torque : Inport
  C&V custom friction : fl_lib/Mechanical/Rotational Elements/Mechanical Rotational Reference
  C&V friction2 : fl_lib/Mechanical/Rotational Elements/Rotational Friction  brkwy_trq=0.4 N*m  brkwy_vel=0.1 rad/s  Col_trq=Bf_plus N*m  visc_coef=0 N*m*s/rad  w_specify=off  w_priority=None  w=0 rad/s  w_nominal_specify=off  w_nominal_unit=rad/s  w_nominal_value=1  t_specify=off  t_priority=None  t=0 N*m  t_nominal_specify=off  t_nominal_unit=N*m  t_nominal_value=1
  Custom Spring : Subsystem
      mask Display: image('C:\Users\laura\OneDrive\Desktop\download.jpeg'); % Use "Edit Image" on toolstrip to change.
  Gear Box : fl_lib/Mechanical/Mechanisms/Gear Box  ratio=N  t_in_specify=off  t_in_priority=None  t_in=0 N*m  t_in_nominal_specify=off  t_in_nominal_unit=N*m  t_in_nominal_value=1  t_out_specify=off  t_out_priority=None  t_out=0 N*m  t_out_nominal_specify=off  t_out_nominal_unit=N*m  t_out_nominal_value=1
  Ideal Rotational Motion Sensor2 : fl_lib/Mechanical/Mechanical Sensors/Ideal Rotational Motion Sensor  reference=foundation.enum.MeasurementReference.absolute  acceleration_port=false  velocity_port=true  position_port=true  wrap_angle=false  offset=0 rad
      settings: InternalSimscapePortConfiguration="{\"Bottom\":[],\"Left\":[{\"id\":\"R\",\"label\":\"R\",\"type\":\"foundation.mechanical.rotational.rotational\"}],\"Right\":[{\"id\":\"W\",\"label\":\"W\",\"type\":\"output\"},{\"id\":\"A\",\"label\":\"A\",\"type\":\"output\"}],\"Top\":[]}"
  Ideal Torque Source : fl_lib/Mechanical/Mechanical Sources/Ideal Torque Source
  Inertia : fl_lib/Mechanical/Rotational Elements/Inertia  inertia=Jin_20 kg*m^2  num_ports=foundation.enum.numPorts2.one  w_specify=off  w_priority=High  w=0 rad/s  w_nominal_specify=off  w_nominal_unit=rad/s  w_nominal_value=1  t_specify=off  t_priority=None  t=0 N*m  t_nominal_specify=off  t_nominal_unit=N*m  t_nominal_value=1
  Mechanical Rotational Reference : fl_lib/Mechanical/Rotational Elements/Mechanical Rotational Reference
  Mechanical Rotational Reference3 : fl_lib/Mechanical/Rotational Elements/Mechanical Rotational Reference
  Mechanical Rotational Reference4 : fl_lib/Mechanical/Rotational Elements/Mechanical Rotational Reference
  PS-Simulink Converter1 : nesl_utility/PS-Simulink Converter  PhysicalDomain=network_engine_domain  SubClassName=ps_output  LeftPortType=input  RightPortType=output  PseudoPeriodic=off  Frequencies=[]  VectorFormat=inherit  Unit=inherit  AffineConversion=off
  PS-Simulink Converter4 : nesl_utility/PS-Simulink Converter  PhysicalDomain=network_engine_domain  SubClassName=ps_output  LeftPortType=input  RightPortType=output  PseudoPeriodic=off  Frequencies=[]  VectorFormat=inherit  Unit=inherit  AffineConversion=off
  Rotational Branch : MyComponent_lib/Rotational Branch  brkwy_trq=25 N*m  brkwy_vel=0.1 rad/s  Col_trq_p=0.008 N*m  Col_trq_m=-0.007 N*m  visc_coef=6.4e-4 N*m*s/rad  w_specify=off  w_priority=None  w=0 rad/s  w_nominal_specify=off  w_nominal_unit=rad/s  w_nominal_value=1  t_specify=off  t_priority=None  t=0 N*m  t_nominal_specify=off  t_nominal_unit=N*m  t_nominal_value=1
      settings: InternalSimscapePortConfiguration="{\"Bottom\":[],\"Left\":[{\"id\":\"R\",\"label\":\"R\",\"type\":\"foundation.mechanical.rotational.rotational\"}],\"Right\":[{\"id\":\"C\",\"label\":\"C\",\"type\":\"foundation.mechanical.rotational.rotational\"}],\"Top\":[]}"
  Rotational Multibody Interface : fl_lib/Mechanical/Multibody Interfaces/Rotational Multibody Interface
  Simulink-PS Converter1 : nesl_utility/Simulink-PS Converter  PhysicalDomain=network_engine_domain  SubClassName=ps_input  LeftPortType=input  RightPortType=output  PseudoPeriodic=off  Frequencies=[]  NoiseDistribution=none  NoiseParameters=[]  Unit=1  AffineConversion=off  FilteringAndDerivatives=provide  SimscapeFilterOrder=1  InputFilterTimeConstant=0.001  UdotUserProvided=0
  torque : PMIOPort  Side=Left
  velocity : PMIOPort  Port=2  Side=Right
  tag scope: dqw2=global, qw2=global
  wires:
  Motor torque/1 -> Simulink-PS Converter1/1
  PS-Simulink Converter1/1 -> [dqw2]
  PS-Simulink Converter4/1 -> [qw2]
  connections:
  Simulink-PS Converter1/RConn1 -- Ideal Torque Source/RConn1
  Mechanical Rotational Reference/LConn1 -- Ideal Torque Source/RConn2
  Rotational Branch/LConn1 -- Ideal Torque Source/LConn1 -- Inertia/LConn1 -- Gear Box/LConn1 -- Ideal Rotational Motion Sensor2/LConn1
  velocity/RConn1 -- Rotational Multibody Interface/RConn1
  torque/RConn1 -- Rotational Multibody Interface/LConn1
  Gear Box/RConn1 -- Custom Spring/LConn1
  Ideal Rotational Motion Sensor2/RConn2 -- PS-Simulink Converter4/LConn1
  Ideal Rotational Motion Sensor2/RConn1 -- PS-Simulink Converter1/LConn1
  Mechanical Rotational Reference3/LConn1 -- Rotational Multibody Interface/LConn2
  Custom Spring/RConn1 -- C&V friction2/LConn1 -- Rotational Multibody Interface/RConn2
  Mechanical Rotational Reference4/LConn1 -- C&V friction2/RConn1
  Rotational Branch/RConn1 -- C&V custom friction/LConn1

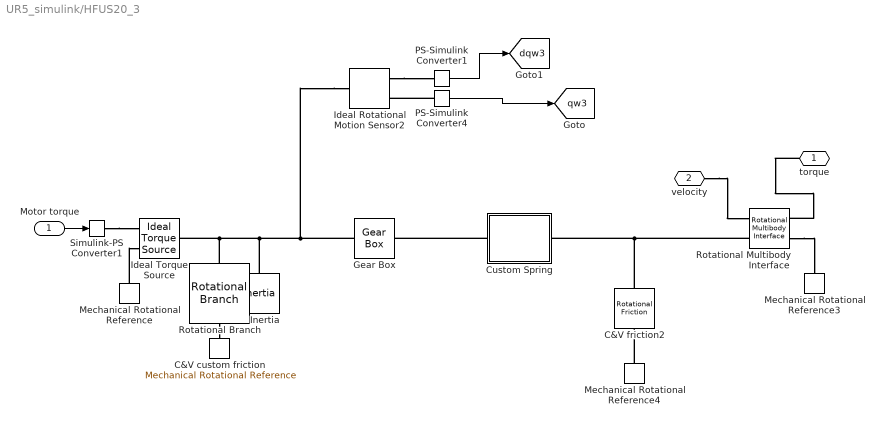
== system UR5_simulink/HFUS20_3 ==
  Motor torque : Inport
  C&V custom friction : fl_lib/Mechanical/Rotational Elements/Mechanical Rotational Reference
  C&V friction2 : fl_lib/Mechanical/Rotational Elements/Rotational Friction  brkwy_trq=0.4 N*m  brkwy_vel=0.1 rad/s  Col_trq=Bf_plus N*m  visc_coef=0 N*m*s/rad  w_specify=off  w_priority=None  w=0 rad/s  w_nominal_specify=off  w_nominal_unit=rad/s  w_nominal_value=1  t_specify=off  t_priority=None  t=0 N*m  t_nominal_specify=off  t_nominal_unit=N*m  t_nominal_value=1
  Custom Spring : Subsystem
      mask Display: image('C:\Users\laura\OneDrive\Desktop\download.jpeg'); % Use "Edit Image" on toolstrip to change.
  Gear Box : fl_lib/Mechanical/Mechanisms/Gear Box  ratio=N  t_in_specify=off  t_in_priority=None  t_in=0 N*m  t_in_nominal_specify=off  t_in_nominal_unit=N*m  t_in_nominal_value=1  t_out_specify=off  t_out_priority=None  t_out=0 N*m  t_out_nominal_specify=off  t_out_nominal_unit=N*m  t_out_nominal_value=1
  Ideal Rotational Motion Sensor2 : fl_lib/Mechanical/Mechanical Sensors/Ideal Rotational Motion Sensor  reference=foundation.enum.MeasurementReference.absolute  acceleration_port=false  velocity_port=true  position_port=true  wrap_angle=false  offset=0 rad
      settings: InternalSimscapePortConfiguration="{\"Bottom\":[],\"Left\":[{\"id\":\"R\",\"label\":\"R\",\"type\":\"foundation.mechanical.rotational.rotational\"}],\"Right\":[{\"id\":\"W\",\"label\":\"W\",\"type\":\"output\"},{\"id\":\"A\",\"label\":\"A\",\"type\":\"output\"}],\"Top\":[]}"
  Ideal Torque Source : fl_lib/Mechanical/Mechanical Sources/Ideal Torque Source
  Inertia : fl_lib/Mechanical/Rotational Elements/Inertia  inertia=Jin_20 kg*m^2  num_ports=foundation.enum.numPorts2.one  w_specify=off  w_priority=High  w=0 rad/s  w_nominal_specify=off  w_nominal_unit=rad/s  w_nominal_value=1  t_specify=off  t_priority=None  t=0 N*m  t_nominal_specify=off  t_nominal_unit=N*m  t_nominal_value=1
  Mechanical Rotational Reference : fl_lib/Mechanical/Rotational Elements/Mechanical Rotational Reference
  Mechanical Rotational Reference3 : fl_lib/Mechanical/Rotational Elements/Mechanical Rotational Reference
  Mechanical Rotational Reference4 : fl_lib/Mechanical/Rotational Elements/Mechanical Rotational Reference
  PS-Simulink Converter1 : nesl_utility/PS-Simulink Converter  PhysicalDomain=network_engine_domain  SubClassName=ps_output  LeftPortType=input  RightPortType=output  PseudoPeriodic=off  Frequencies=[]  VectorFormat=inherit  Unit=inherit  AffineConversion=off
  PS-Simulink Converter4 : nesl_utility/PS-Simulink Converter  PhysicalDomain=network_engine_domain  SubClassName=ps_output  LeftPortType=input  RightPortType=output  PseudoPeriodic=off  Frequencies=[]  VectorFormat=inherit  Unit=inherit  AffineConversion=off
  Rotational Branch : MyComponent_lib/Rotational Branch  brkwy_trq=25 N*m  brkwy_vel=0.1 rad/s  Col_trq_p=0.008 N*m  Col_trq_m=-0.007 N*m  visc_coef=6.4e-4 N*m*s/rad  w_specify=off  w_priority=None  w=0 rad/s  w_nominal_specify=off  w_nominal_unit=rad/s  w_nominal_value=1  t_specify=off  t_priority=None  t=0 N*m  t_nominal_specify=off  t_nominal_unit=N*m  t_nominal_value=1
      settings: InternalSimscapePortConfiguration="{\"Bottom\":[],\"Left\":[{\"id\":\"R\",\"label\":\"R\",\"type\":\"foundation.mechanical.rotational.rotational\"}],\"Right\":[{\"id\":\"C\",\"label\":\"C\",\"type\":\"foundation.mechanical.rotational.rotational\"}],\"Top\":[]}"
  Rotational Multibody Interface : fl_lib/Mechanical/Multibody Interfaces/Rotational Multibody Interface
  Simulink-PS Converter1 : nesl_utility/Simulink-PS Converter  PhysicalDomain=network_engine_domain  SubClassName=ps_input  LeftPortType=input  RightPortType=output  PseudoPeriodic=off  Frequencies=[]  NoiseDistribution=none  NoiseParameters=[]  Unit=1  AffineConversion=off  FilteringAndDerivatives=provide  SimscapeFilterOrder=1  InputFilterTimeConstant=0.001  UdotUserProvided=0
  torque : PMIOPort  Side=Left
  velocity : PMIOPort  Port=2  Side=Right
  tag scope: dqw3=global, qw3=global
  wires:
  Motor torque/1 -> Simulink-PS Converter1/1
  PS-Simulink Converter1/1 -> [dqw3]
  PS-Simulink Converter4/1 -> [qw3]
  connections:
  Rotational Multibody Interface/RConn2 -- Custom Spring/RConn1 -- C&V friction2/LConn1
  Simulink-PS Converter1/RConn1 -- Ideal Torque Source/RConn1
  Mechanical Rotational Reference/LConn1 -- Ideal Torque Source/RConn2
  Ideal Rotational Motion Sensor2/LConn1 -- Gear Box/LConn1 -- Inertia/LConn1 -- Rotational Branch/LConn1 -- Ideal Torque Source/LConn1
  velocity/RConn1 -- Rotational Multibody Interface/RConn1
  torque/RConn1 -- Rotational Multibody Interface/LConn1
  Ideal Rotational Motion Sensor2/RConn1 -- PS-Simulink Converter1/LConn1
  PS-Simulink Converter4/LConn1 -- Ideal Rotational Motion Sensor2/RConn2
  Rotational Multibody Interface/LConn2 -- Mechanical Rotational Reference3/LConn1
  Custom Spring/LConn1 -- Gear Box/RConn1
  Mechanical Rotational Reference4/LConn1 -- C&V friction2/RConn1
  Rotational Branch/RConn1 -- C&V custom friction/LConn1
